simulink model "MBD_Enabled_Subsystem"  (R2021b)
settings: Solver=FixedStepDiscrete  StartTime=0.0  StopTime=10.0  FixedStep=0.001  RelTol=1e-3
libraries: simulink x1
settings Model: Creator=waleed.elshemy  LastModifiedBy=waleed.elshemy
settings OptimizationCC: DefaultParameterBehavior=Inlined  UseDivisionForNetSlopeComputation=on  GainParamInheritBuiltInType=on  UseFloatMulNetSlope=on  InlineInvariantSignals=on  PassReuseOutputArgsAs=Individual arguments  ZeroExternalMemoryAtStartup=off  ZeroInternalMemoryAtStartup=off  NoFixptDivByZeroProtection=on  EfficientFloat2IntCast=on  LifeSpan=1  OptimizeBlockOrder=speed  DifferentSizesBufferReuse=on  EfficientTunableParamExpr=on
settings DebuggingCC: ParameterTunabilityLossMsg=error
settings HardwareCC: ProdLongLongMode=on
settings SFSimCC: MATLABDynamicMemAlloc=off
settings RTWCC: Description=Embedded Coder  SystemTargetFile=ert.tlc  TemplateMakefile=ert_default_tmf
settings CodeAppCC: ForceParamTrailComments=on  IgnoreCustomStorageClasses=off  OperatorAnnotations=on  SimulinkDataObjDesc=on  SFDataObjDesc=on  CustomSymbolStrGlobalVar=rt$N$M  CustomSymbolStrType=$N$M  CustomSymbolStrFcn=$N$M$F  CustomSymbolStrMacro=$N$M  InsertBlockDesc=on
settings ERTTargetCC: TargetLangStandard=C99 (ISO)  GenerateSampleERTMain=on  IncludeMdlTerminateFcn=off  CombineSignalStateStructs=on  SupportComplex=off  SupportContinuousTime=on  InlinedParameterPlacement=NonHierarchical  ERTCustomFileTemplate=example_file_process.tlc

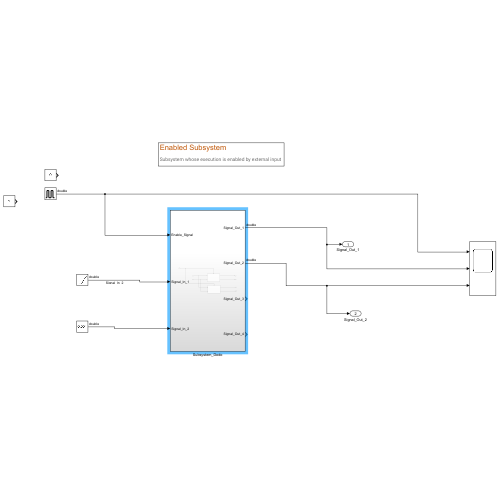
[thumbnail: Simulink's stored preview of the top-level diagram]
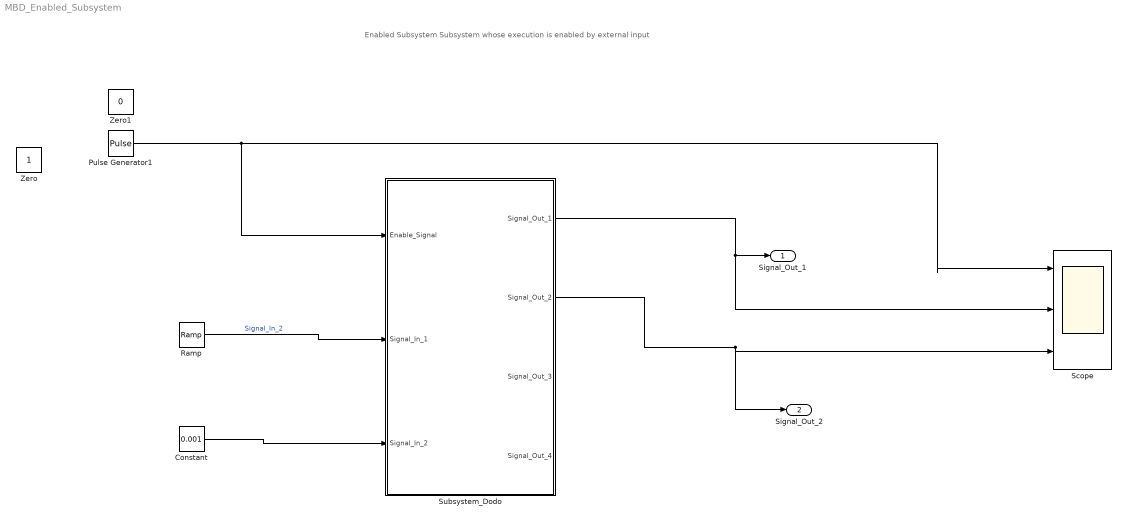
== system MBD_Enabled_Subsystem ==
  note: Enabled Subsystem
      | Subsystem whose execution is enabled by external input
  Constant : Constant  Value=0.001
  Pulse Generator1 : DiscretePulseGenerator  PulseType=Time based  Period=7  PulseWidth=50
  Ramp : simulink/Sources/Ramp  slope=0.01  start=0  InitialOutput=0
  Scope : Scope  NumInputPorts=3
  Subsystem_Dodo : Subsystem
  Zero : Constant  OutDataTypeStr=Inherit: Inherit via back propagation
  Zero1 : Constant  Value=0  OutDataTypeStr=Inherit: Inherit via back propagation
  Signal_Out_1 : Outport
  Signal_Out_2 : Outport  Port=2
  wires:
  Ramp/1 -> Subsystem_Dodo/2(Signal_In_1)  "Signal_In_2"
  Subsystem_Dodo/1(Signal_Out_1) -> Scope/2, Signal_Out_1/1
  Subsystem_Dodo/2(Signal_Out_2) -> Signal_Out_2/1, Scope/3
  Pulse Generator1/1 -> Subsystem_Dodo/1(Enable_Signal), Scope/1
  Constant/1 -> Subsystem_Dodo/3(Signal_In_2)

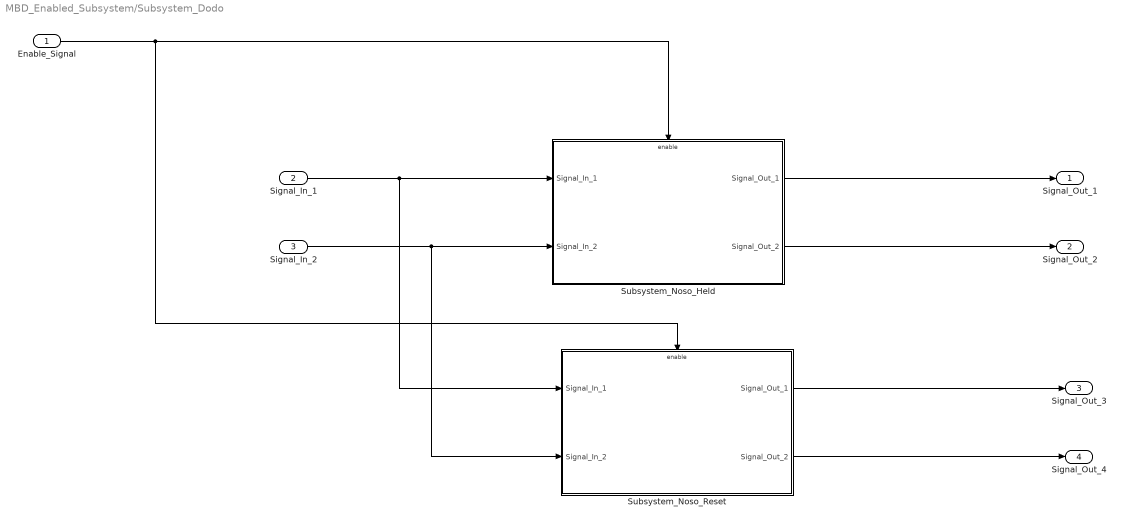
== system MBD_Enabled_Subsystem/Subsystem_Dodo ==
  Enable_Signal : Inport
  Signal_In_1 : Inport  Port=2
  Signal_In_2 : Inport  Port=3
  Subsystem_Noso_Held : Subsystem  TreatAsAtomicUnit=on
  Subsystem_Noso_Reset : Subsystem  TreatAsAtomicUnit=on
      settings: RTWFileNameOpts=Use function name
  Signal_Out_1 : Outport
  Signal_Out_2 : Outport  Port=2
  Signal_Out_3 : Outport  Port=3
  Signal_Out_4 : Outport  Port=4
  wires:
  Subsystem_Noso_Held/1(Signal_Out_1) -> Signal_Out_1/1
  Signal_In_1/1 -> Subsystem_Noso_Reset/1(Signal_In_1), Subsystem_Noso_Held/1(Signal_In_1)
  Signal_In_2/1 -> Subsystem_Noso_Reset/2(Signal_In_2), Subsystem_Noso_Held/2(Signal_In_2)
  Subsystem_Noso_Held/2(Signal_Out_2) -> Signal_Out_2/1
  Enable_Signal/1 -> Subsystem_Noso_Held/Enable, Subsystem_Noso_Reset/Enable
  Subsystem_Noso_Reset/1(Signal_Out_1) -> Signal_Out_3/1
  Subsystem_Noso_Reset/2(Signal_Out_2) -> Signal_Out_4/1

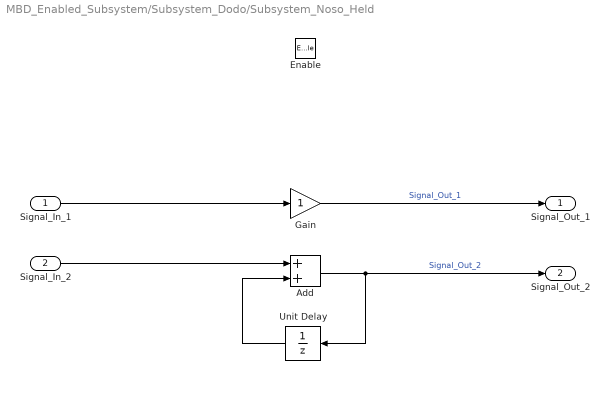
== system MBD_Enabled_Subsystem/Subsystem_Dodo/Subsystem_Noso_Held ==
  Signal_In_1 : Inport
  Signal_In_2 : Inport  Port=2
  Enable : EnablePort
  Add : Sum
  Gain : Gain
  Unit Delay : UnitDelay  SampleTime=-1  HasFrameUpgradeWarning=on
  Signal_Out_1 : Outport
  Signal_Out_2 : Outport  Port=2
  wires:
  Add/1 -> Signal_Out_2/1, Unit Delay/1  "Signal_Out_2"
  Gain/1 -> Signal_Out_1/1  "Signal_Out_1"
  Signal_In_2/1 -> Add/1
  Unit Delay/1 -> Add/2
  Signal_In_1/1 -> Gain/1

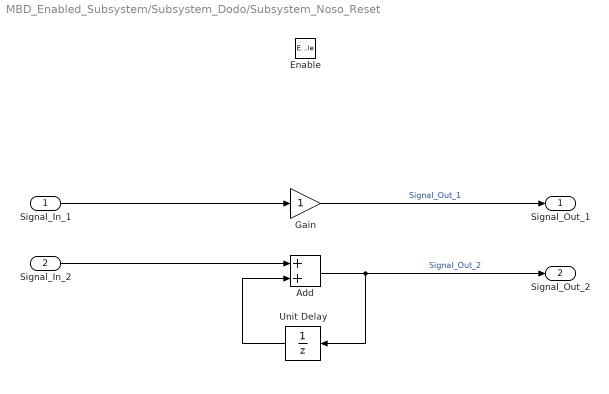
== system MBD_Enabled_Subsystem/Subsystem_Dodo/Subsystem_Noso_Reset ==
  Signal_In_1 : Inport
  Signal_In_2 : Inport  Port=2
  Enable : EnablePort  StatesWhenEnabling=reset
  Add : Sum
  Gain : Gain
  Unit Delay : UnitDelay  SampleTime=-1  HasFrameUpgradeWarning=on
  Signal_Out_1 : Outport
  Signal_Out_2 : Outport  Port=2
  wires:
  Signal_In_1/1 -> Gain/1
  Unit Delay/1 -> Add/2
  Signal_In_2/1 -> Add/1
  Gain/1 -> Signal_Out_1/1  "Signal_Out_1"
  Add/1 -> Unit Delay/1, Signal_Out_2/1  "Signal_Out_2"
